simulink model "highpassderivative"  (R2021a)
settings: Solver=VariableStepAuto  StartTime=0.0  StopTime=10.0  RelTol=1e-3
settings Model: Creator=templ  LastModifiedBy=templ

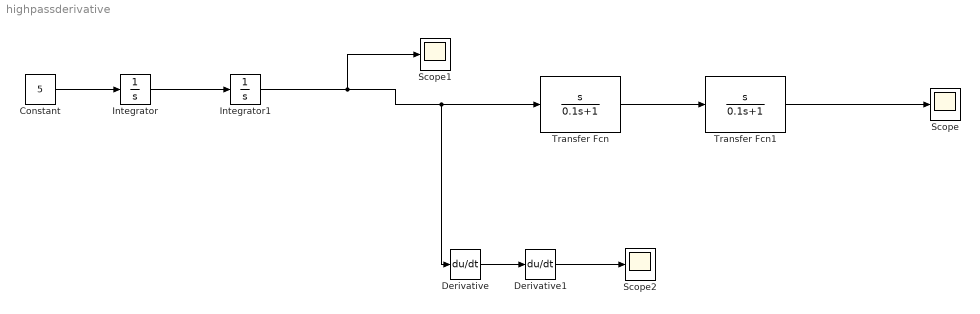
== system highpassderivative ==
  Constant : Constant  Value=5
  Derivative : Derivative  CoefficientInTFapproximation=1
  Derivative1 : Derivative  CoefficientInTFapproximation=1
  Integrator : Integrator
  Integrator1 : Integrator
  Scope : Scope
  Scope1 : Scope
  Scope2 : Scope
  Transfer Fcn : TransferFcn  Numerator=[1 0]  Denominator=[0.1 1]
  Transfer Fcn1 : TransferFcn  Numerator=[1 0]  Denominator=[0.1 1]
  wires:
  Constant/1 -> Integrator/1
  Integrator/1 -> Integrator1/1
  Integrator1/1 -> Scope1/1, Derivative/1, Transfer Fcn/1
  Transfer Fcn/1 -> Transfer Fcn1/1
  Derivative/1 -> Derivative1/1
  Derivative1/1 -> Scope2/1
  Transfer Fcn1/1 -> Scope/1
